simulink model "ARINCFCCD2CU"  (R2021b)
settings: Solver=FixedStepDiscrete  StartTime=0.0  StopTime=2  RelTol=1e-3
undefined symbols (not defined in the file): ACE8_MODE, ACE9_MODE, ACE_ID, ARINC1_ERR, ARINC3_ERR, ARINC5_ERR, ARINC6_ERR, ARINC9_ERR, GEARING_APPLIED, IO682, RAM_POS, RAM_POS_FAILURE, ROLL_POS, ROLL_POS_FAILURE, SPD, SPD_FAILURE
libraries: speedgoatlib_IO682 x13
settings Model: Creator=ACH  LastModifiedBy=angel
settings SolverCC: ConcurrentTasks=on  PositivePriorityOrder=on
settings OptimizationCC: BlockReduction=off  OptimizeBlockIOStorage=off
settings DebuggingCC: TasksWithSamePriorityMsg=none
settings HardwareCC: ProdBitPerLong=64  ProdLongLongMode=on  ProdHWDeviceType=Intel->x86-64 (Linux 64)
settings RTWCC: Description=Simulink Real-Time  SystemTargetFile=slrealtime.tlc  TemplateMakefile=slrealtime_default_tmf  Toolchain=Simulink Real-Time Toolchain  BuildConfiguration=Faster Runs  CodeExecutionProfiling=on  TargetLang=C++
settings SimulinkRealTimeTargetCC: UseGCCFastMath=on

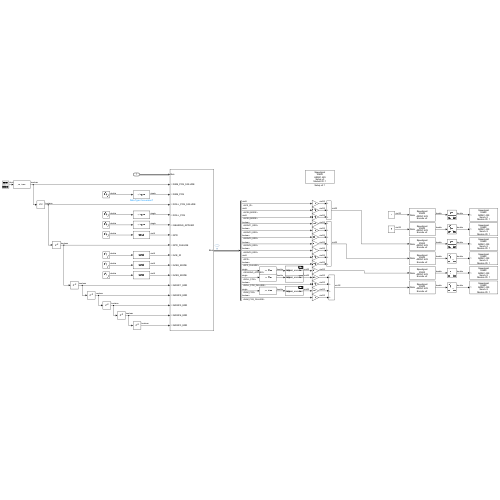
[thumbnail: Simulink's stored preview of the top-level diagram]
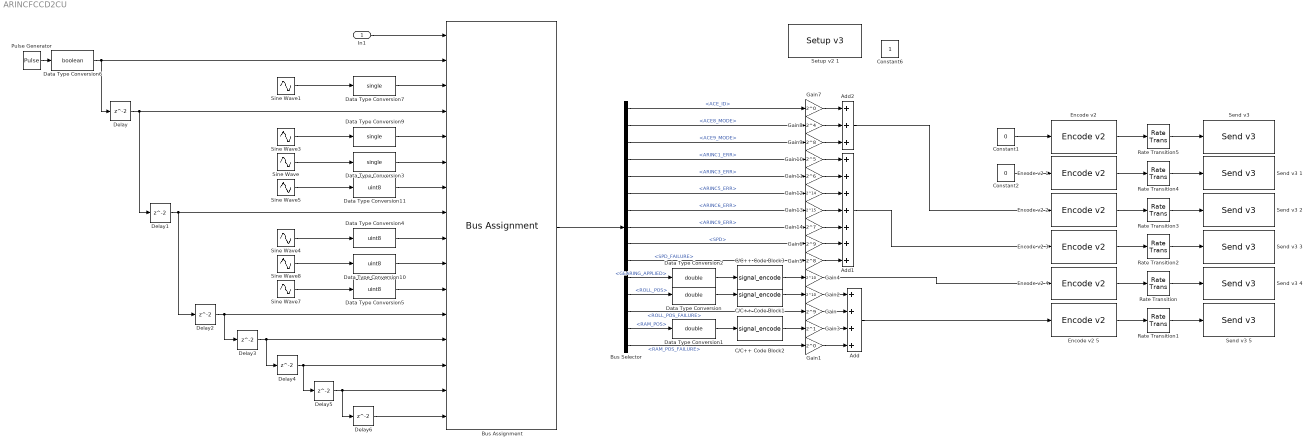
== system ARINCFCCD2CU ==
  In1 : Inport  OutDataTypeStr=Bus: ACE8C_FCC1
  Add : Sum  Inputs=++++
  Add1 : Sum  Inputs=+++++++
  Add2 : Sum  Inputs=+++
  Bus Assignment : BusAssignment  AssignedSignals=RAM_POS_FAILURE,RAM_POS,ROLL_POS_FAILURE,ROLL_POS,GEARING_APPLIED,SPD,SPD_FAILURE,ACE_ID,ACE8_MODE,ACE9_MODE,ARINC1_ERR,ARINC9_ERR,ARINC5_ERR,ARINC6_ERR,ARINC3_ERR
  Bus Selector : BusSelector  OutputSignals=ACE_ID,ACE8_MODE,ACE9_MODE,ARINC1_ERR,ARINC3_ERR,ARINC5_ERR,ARINC6_ERR,ARINC9_ERR,SPD,SPD_FAILURE,GEARING_APPLIED,ROLL_POS,ROLL_POS_FAILURE,RAM_POS,RAM_POS_FAILURE
  C/C++ Code Block1 : S-Function  FunctionName=signal_encode  Parameters=6.29921E-1,0,boolean(1),boolean(0),uint32(8)  SFunctionModules=signal_encode_wrapper  SFunctionDeploymentMode=off  EnableBusSupport=off  mask(S-Function Builder){}
      mask help: Simulink:masks:SFunctionBuilder_MD
      mask init:
      | val = [[.9  0.75 0.75 1 1 .9 .9 1]',[1 1 0.75 0.75 .9 .9 1 .9]'];try , sys = get_param(gcb,'SfunBuilderFcnName');if isempty(sys), sys = get_param(gcb,'FunctionName'); end,catch, sys = get_param(gcb,'FunctionName'); end
      settings: CopyFcn=set_param(gcbh,'LinkStatus','none')  OpenFcn=sfunctionwizard(gcbh)
      mask Display:
      | plot(val(:,1),val(:,2))
      | disp(sys)
      | port_label('input',1,'data')
      | port_label('output',1,'out')
  C/C++ Code Block2 : S-Function  FunctionName=signal_encode  Parameters=2.12598E-1,0,boolean(1),boolean(0),uint32(8)  SFunctionModules=signal_encode_wrapper  SFunctionDeploymentMode=off  EnableBusSupport=off  mask(S-Function Builder){}
      mask help: Simulink:masks:SFunctionBuilder_MD
      mask init: same as ARINCFCCD2CU/C/C++ Code Block1
      settings: CopyFcn=set_param(gcbh,'LinkStatus','none')  OpenFcn=sfunctionwizard(gcbh)
      mask Display:
      | plot(val(:,1),val(:,2))
      | disp(sys)
      | port_label('input',1,'data')
      | port_label('output',1,'out')
  C/C++ Code Block3 : S-Function  FunctionName=signal_encode  Parameters=1.96851E-3,0.2,boolean(0),boolean(0),uint32(7)  SFunctionModules=signal_encode_wrapper  SFunctionDeploymentMode=off  EnableBusSupport=off  mask(S-Function Builder){}
      mask help: Simulink:masks:SFunctionBuilder_MD
      mask init: same as ARINCFCCD2CU/C/C++ Code Block1
      settings: CopyFcn=set_param(gcbh,'LinkStatus','none')  OpenFcn=sfunctionwizard(gcbh)
      mask Display:
      | plot(val(:,1),val(:,2))
      | disp(sys)
      | port_label('input',1,'data')
      | port_label('output',1,'out')
  Constant1 : Constant  Value=0  OutDataTypeStr=uint32
  Constant2 : Constant  Value=0  OutDataTypeStr=uint32
  Data Type Conversion : DataTypeConversion  OutDataTypeStr=double
  Data Type Conversion1 : DataTypeConversion  OutDataTypeStr=double
  Data Type Conversion{4..5,10..11} (4 alike) : DataTypeConversion  OutDataTypeStr=uint8
  Data Type Conversion2 : DataTypeConversion  OutDataTypeStr=double
  Data Type Conversion3 : DataTypeConversion  OutDataTypeStr=single
  Data Type Conversion6 : DataTypeConversion  OutDataTypeStr=boolean
  Data Type Conversion7 : DataTypeConversion  OutDataTypeStr=single
  Data Type Conversion9 : DataTypeConversion  OutDataTypeStr=single
  Delay{,1..6} (7 alike) : Delay
  "Encode v2 " : speedgoatlib_IO682/Encode v2   parMode=Custom Data Type  parLabel=[55]  parDataType=[0]  parResolution=[1]  parBits=[19]  parSdi=[0]  parSsm=[-1]  parCustomDataType=Raw  parDataLSB=11  parDataMSB=31  parBitPosition=[9, 31]  parScaleBNR=1  parExponent=8  parMantissa=14  parEnSSM=off
      settings: SourceProductName=Simulink Real-Time: Speedgoat I/O Blockset
  Encode v2 1 : speedgoatlib_IO682/Encode v2   parMode=Custom Data Type  parLabel=[305]  parDataType=[0]  parResolution=[1]  parBits=[19]  parSdi=[0]  parSsm=[-1]  parCustomDataType=Raw  parDataLSB=11  parDataMSB=31  parBitPosition=[9, 31]  parScaleBNR=1  parExponent=8  parMantissa=14  parEnSSM=off
      settings: SourceProductName=Simulink Real-Time: Speedgoat I/O Blockset
  Encode v2 2 : speedgoatlib_IO682/Encode v2   parMode=Custom Data Type  parLabel=[112]  parDataType=[0]  parResolution=[1]  parBits=[19]  parSdi=[0]  parSsm=[-1]  parCustomDataType=Raw  parDataLSB=11  parDataMSB=31  parBitPosition=[9, 31]  parScaleBNR=1  parExponent=8  parMantissa=14  parEnSSM=off
      settings: SourceProductName=Simulink Real-Time: Speedgoat I/O Blockset
  Encode v2 3 : speedgoatlib_IO682/Encode v2   parMode=Custom Data Type  parLabel=[163]  parDataType=[0]  parResolution=[1]  parBits=[19]  parSdi=[0]  parSsm=[-1]  parCustomDataType=Raw  parDataLSB=11  parDataMSB=31  parBitPosition=[9, 31]  parScaleBNR=1  parExponent=8  parMantissa=14  parEnSSM=off
      settings: SourceProductName=Simulink Real-Time: Speedgoat I/O Blockset
  Encode v2 4 : speedgoatlib_IO682/Encode v2   parMode=Custom Data Type  parLabel=[231]  parDataType=[0]  parResolution=[1]  parBits=[19]  parSdi=[0]  parSsm=[-1]  parCustomDataType=Raw  parDataLSB=11  parDataMSB=31  parBitPosition=[9, 31]  parScaleBNR=1  parExponent=8  parMantissa=14  parEnSSM=off
      settings: SourceProductName=Simulink Real-Time: Speedgoat I/O Blockset
  Encode v2 5 : speedgoatlib_IO682/Encode v2   parMode=Custom Data Type  parLabel=[265]  parDataType=[0]  parResolution=[1]  parBits=[19]  parSdi=[0]  parSsm=[-1]  parCustomDataType=Raw  parDataLSB=11  parDataMSB=31  parBitPosition=[9, 31]  parScaleBNR=1  parExponent=8  parMantissa=14  parEnSSM=off
      settings: SourceProductName=Simulink Real-Time: Speedgoat I/O Blockset
  Gain : Gain  Gain=2^9  OutDataTypeStr=uint32
  Gain1 : Gain  Gain=2^0  OutDataTypeStr=uint32
  Gain10 : Gain  Gain=2^5  OutDataTypeStr=uint32
  Gain11 : Gain  Gain=2^6  OutDataTypeStr=uint32
  Gain12 : Gain  Gain=2^14  OutDataTypeStr=uint32
  Gain13 : Gain  Gain=2^15  OutDataTypeStr=uint32
  Gain14 : Gain  Gain=2^7  OutDataTypeStr=uint32
  Gain2 : Gain  Gain=2^10  OutDataTypeStr=uint32
  Gain3 : Gain  Gain=2^1  OutDataTypeStr=uint32
  Gain4 : Gain  Gain=2^10  OutDataTypeStr=uint32
  Gain5 : Gain  Gain=2^8  OutDataTypeStr=uint32
  Gain6 : Gain  Gain=2^9  OutDataTypeStr=uint32
  Gain7 : Gain  Gain=2^0  OutDataTypeStr=uint32
  Gain8 : Gain  Gain=2^4  OutDataTypeStr=uint32
  Gain9 : Gain  Gain=2^8  OutDataTypeStr=uint32
  Pulse Generator : DiscretePulseGenerator  Period=125  PulseWidth=25  SampleTime=0.008
  Rate Transition{,1..5} (6 alike) : RateTransition
  "Send v3 " : speedgoatlib_IO682/Send v3   parModuleId=1  parChannel=1  parSampleTime=0.064
      settings: SourceProductName=Simulink Real-Time: Speedgoat I/O Blockset
  Send v3 1 : speedgoatlib_IO682/Send v3   parModuleId=1  parChannel=1  parSampleTime=0.064
      settings: SourceProductName=Simulink Real-Time: Speedgoat I/O Blockset
  Send v3 {2..5} (4 alike) : speedgoatlib_IO682/Send v3   parModuleId=1  parChannel=1  parSampleTime=0.016
      settings: SourceProductName=Simulink Real-Time: Speedgoat I/O Blockset
  Setup v2 1 : speedgoatlib_IO682/Setup v3   parModuleId=1  parBoardVariant=IO682-16-16  parPciSlot=-1  parTimerCount=4000*8  parChannelMode=Manual  parInBitRate1=100000  parInBufferMode1=Individual  parInEnable1=on  parInParity1=off  parInInternalWrap1=off  parInBitRate2=100000  parInBufferMode2=Individual  parInEnable2=on  parInParity2=on  parInInternalWrap2=off  parInBitRate3=100000  parInBufferMode3=Individual  parInEnable3=on  parInParity3=on  parInInternalWrap3=off  parInBitRate4=100000  parInBufferMode4=Individual  parInEnable4=on  parInParity4=on  parInInternalWrap4=off  parInBitRate5=100000  parInBufferMode5=Individual  parInEnable5=on  parInParity5=on  parInInternalWrap5=off  parInBitRate6=100000  parInBufferMode6=Individual  parInEnable6=on  parInParity6=on  parInInternalWrap6=off  parInBitRate7=100000  parInBufferMode7=Individual  parInEnable7=on  parInParity7=on  parInInternalWrap7=off  parInBitRate8=100000  parInBufferMode8=Individual  parInEnable8=on  parInParity8=on  parInInternalWrap8=off  parInBitRate9=100000  parInBufferMode9=Individual  parInEnable9=on  parInParity9=on  parInInternalWrap9=off  parInBitRate10=100000  parInBufferMode10=Individual  parInEnable10=on  parInParity10=on  parInInternalWrap10=off  parInBitRate11=100000  parInBufferMode11=Individual  parInEnable11=on  parInParity11=on  parInInternalWrap11=off  parInBitRate12=100000  parInBufferMode12=Individual  parInEnable12=on  parInParity12=on  parInInternalWrap12=off  parInBitRate13=100000  parInBufferMode13=Individual  parInEnable13=on  parInParity13=on  parInInternalWrap13=off  parInBitRate14=100000  parInBufferMode14=Individual  parInEnable14=on  parInParity14=on  parInInternalWrap14=off  parInBitRate15=100000  parInBufferMode15=Individual  parInEnable15=on  parInParity15=on  parInInternalWrap15=off  parInBitRate16=100000  parInBufferMode16=Individual  parInEnable16=on  parInParity16=on  parInInternalWrap16=off  parOutBitRate1=100000  parOutParity1=Odd  parOutProtocolError1=None  parOutEnable1=on  parOutBitRate2=100000  parOutParity2=Odd  parOutProtocolError2=None  parOutEnable2=on  parOutBitRate3=100000  parOutParity3=Odd  parOutProtocolError3=None  parOutEnable3=on  parOutBitRate4=100000  parOutParity4=Odd  parOutProtocolError4=None  parOutEnable4=on  parOutBitRate5=100000  parOutParity5=Odd  parOutProtocolError5=None  parOutEnable5=on  parOutBitRate6=100000  parOutParity6=Odd  parOutProtocolError6=None  parOutEnable6=on  parOutBitRate7=100000  parOutParity7=Odd  parOutProtocolError7=None  parOutEnable7=on  parOutBitRate8=100000  parOutParity8=Odd  parOutProtocolError8=None  parOutEnable8=on  parOutBitRate9=100000  parOutParity9=Odd  parOutProtocolError9=None  parOutEnable9=on  parOutBitRate10=100000  parOutParity10=Odd  parOutProtocolError10=None  parOutEnable10=on  parOutBitRate11=100000  parOutParity11=Odd  parOutProtocolError11=None  parOutEnable11=on  parOutBitRate12=100000  parOutParity12=Odd  parOutProtocolError12=None  parOutEnable12=on  parOutBitRate13=100000  parOutParity13=Odd  parOutProtocolError13=None  parOutEnable13=on  parOutBitRate14=100000  parOutParity14=Odd  parOutProtocolError14=None  parOutEnable14=on  parOutBitRate15=100000  parOutParity15=Odd  parOutProtocolError15=None  parOutEnable15=on  parOutBitRate16=100000  parOutParity16=Odd  parOutProtocolError16=None  parOutEnable16=on  parChConfigFile=''  parScheduleMode=Manual  parScheduledMsgConfigFile=''  parHwDeviceId=hex2dec('0830')  parTimeSource=Internal timer  parChInConfig=[158 8 7 8 1;158 8 7 7 1;158 8 7 7 1;158 8 7 7 1;158 8 7 7 1;158 8 7 7 1;158 8 7 7 1;158 8 7 7 1;158 8 7 7 1;158 8 7 7 1;158 8 7 7 1;158 8 7 7 1;158 8 7 7 1;158 8 7 7 1;158 8 7 7 1;158 8 7 7 1]  parChOutConfig=[158 0 4 7;158 0 4 7;158 0 4 7;158 0 4 7;158 0 4 7;158 0 4 7;158 0 4 7;158 0 4 7;158 0 4 7;158 0 4 7;158 0 4 7;158 0 4 7;158 0 4 7;158 0 4 7;158 0 4 7;158 0 4 7]  parScheduledMessages=0
      settings: SourceProductName=Speedgoat I/O Blockset
  Sine Wave : Sin  Amplitude=(0.45-0.2)/2*0.99  Bias=0.2+(0.45-0.2)/2  Frequency=2*pi  SampleTime=0.008
  Sine Wave1 : Sin  Amplitude=27*0.99  Frequency=2*pi  SampleTime=0.008
  Sine Wave3 : Sin  Amplitude=80*0.99  Frequency=2*pi  SampleTime=0.008
  Sine Wave4 : Sin  Amplitude=7.5  Bias=8  Frequency=2*pi  SampleTime=0.008
  Sine Wave5 : Sin  Amplitude=1.5  Bias=2  Frequency=2*pi  SampleTime=0.008
  Sine Wave7 : Sin  Amplitude=3.5  Bias=4  Frequency=2*pi  SampleTime=0.008
  Sine Wave8 : Sin  Amplitude=3.5  Bias=4  Frequency=2*pi  Phase=pi  SampleTime=0.008
  Constant6 : Constant  IOType=siggen
  wires:
  Constant1/1 -> "Encode v2 "/1
  Encode v2 1/1 -> Rate Transition4/1
  Constant2/1 -> Encode v2 1/1
  Encode v2 2/1 -> Rate Transition3/1
  Encode v2 3/1 -> Rate Transition2/1
  Encode v2 4/1 -> Rate Transition/1
  Encode v2 5/1 -> Rate Transition1/1
  Add2/1 -> Encode v2 2/1
  Add1/1 -> Encode v2 3/1
  Gain4/1 -> Encode v2 4/1
  Add/1 -> Encode v2 5/1
  Bus Assignment/1 -> Bus Selector/1
  Bus Selector/15 -> Gain1/1  "<RAM_POS_FAILURE>"
  Bus Selector/14 -> Data Type Conversion1/1  "<RAM_POS>"
  Bus Selector/13 -> Gain/1  "<ROLL_POS_FAILURE>"
  Bus Selector/12 -> Data Type Conversion/1  "<ROLL_POS>"
  C/C++ Code Block2/1 -> Gain3/1
  C/C++ Code Block1/1 -> Gain2/1
  Gain2/1 -> Add/1
  Gain/1 -> Add/2
  Gain3/1 -> Add/3
  Gain1/1 -> Add/4
  Data Type Conversion/1 -> C/C++ Code Block1/1
  Data Type Conversion1/1 -> C/C++ Code Block2/1
  In1/1 -> Bus Assignment/1
  Bus Selector/11 -> Data Type Conversion2/1  "<GEARING_APPLIED>"
  Data Type Conversion2/1 -> C/C++ Code Block3/1
  C/C++ Code Block3/1 -> Gain4/1
  Bus Selector/9 -> Gain6/1  "<SPD>"
  Bus Selector/10 -> Gain5/1  "<SPD_FAILURE>"
  Gain5/1 -> Add1/7
  Gain6/1 -> Add1/6
  Bus Selector/1 -> Gain7/1  "<ACE_ID>"
  Bus Selector/2 -> Gain8/1  "<ACE8_MODE>"
  Bus Selector/3 -> Gain9/1  "<ACE9_MODE>"
  Gain7/1 -> Add2/1
  Gain8/1 -> Add2/2
  Gain9/1 -> Add2/3
  "Encode v2 "/1 -> Rate Transition5/1
  Data Type Conversion9/1 -> Bus Assignment/5
  Data Type Conversion6/1 -> Delay/1, Bus Assignment/2
  Sine Wave3/1 -> Data Type Conversion9/1
  Sine Wave/1 -> Data Type Conversion3/1
  Delay/1 -> Delay1/1, Bus Assignment/4
  Sine Wave1/1 -> Data Type Conversion7/1
  Pulse Generator/1 -> Data Type Conversion6/1
  Data Type Conversion7/1 -> Bus Assignment/3
  Data Type Conversion3/1 -> Bus Assignment/6
  Sine Wave5/1 -> Data Type Conversion11/1
  Data Type Conversion11/1 -> Bus Assignment/7
  Sine Wave4/1 -> Data Type Conversion4/1
  Data Type Conversion4/1 -> Bus Assignment/9
  Data Type Conversion5/1 -> Bus Assignment/11
  Sine Wave7/1 -> Data Type Conversion5/1
  Sine Wave8/1 -> Data Type Conversion10/1
  Data Type Conversion10/1 -> Bus Assignment/10
  Delay1/1 -> Delay2/1, Bus Assignment/8
  Delay2/1 -> Delay3/1, Bus Assignment/12
  Delay3/1 -> Delay4/1, Bus Assignment/13
  Delay4/1 -> Delay5/1, Bus Assignment/14
  Delay5/1 -> Delay6/1, Bus Assignment/15
  Delay6/1 -> Bus Assignment/16
  Bus Selector/4 -> Gain10/1  "<ARINC1_ERR>"
  Bus Selector/5 -> Gain11/1  "<ARINC3_ERR>"
  Bus Selector/6 -> Gain12/1  "<ARINC5_ERR>"
  Bus Selector/7 -> Gain13/1  "<ARINC6_ERR>"
  Bus Selector/8 -> Gain14/1  "<ARINC9_ERR>"
  Gain10/1 -> Add1/1
  Gain11/1 -> Add1/2
  Gain12/1 -> Add1/3
  Gain13/1 -> Add1/4
  Gain14/1 -> Add1/5
  Rate Transition/1 -> Send v3 4/1
  Rate Transition1/1 -> Send v3 5/1
  Rate Transition2/1 -> Send v3 3/1
  Rate Transition3/1 -> Send v3 2/1
  Rate Transition4/1 -> Send v3 1/1
  Rate Transition5/1 -> "Send v3 "/1
